simulink model "traiettoria"  (R2022b)
settings: Solver=VariableStepAuto  StartTime=0.0  StopTime=40  RelTol=1e-3
values from neighbouring files (symbols this model uses):
  a1 = W \ [0 0 0.5*pi/2 0]'    [traiettoria_script.m]
  a2 = W \ [0 0 0.25 0]'    [traiettoria_script.m]
  a2_phi = W \ [0 0 pi/2 0]'    [traiettoria_script.m]
  a3 = W \ [0 0 0.25 0]'    [traiettoria_script.m]
  a4 = W \ [0 0 0.5*pi/2 0]'    [traiettoria_script.m]
  a5 = W \ [0 0 0.25 0]'    [traiettoria_script.m]
  a6 = W \ [0 0 0.25 0]'    [traiettoria_script.m]
  a6_phi = W \ [0 0 pi/2 0]'    [traiettoria_script.m]
  a7 = W \ [0 0 0.5*pi/2 0]'    [traiettoria_script.m]
  a8 = W \ [0 0 0.5*pi/2 0]'    [traiettoria_script.m]
  a9 = W \ [0 0 (sqrt(5)/4)*(pi - 2*atan(1/2)) 0]'    [traiettoria_script.m]
  p_d_0 = [0 0.75 -0.25]'    [traiettoria_script.m]
  phi_d_0 = 0    [traiettoria_script.m]
  T = T_A * T_B    [DH_dinamica.m]    (also in traiettoria_script.m = 0.001)
undefined symbols (not defined in the file or in its folder): DiscIntNeverNeededParam
settings Model: Creator=Michele  LastModifiedBy=Michele
settings DataIOCC: ReturnWorkspaceOutputs=off

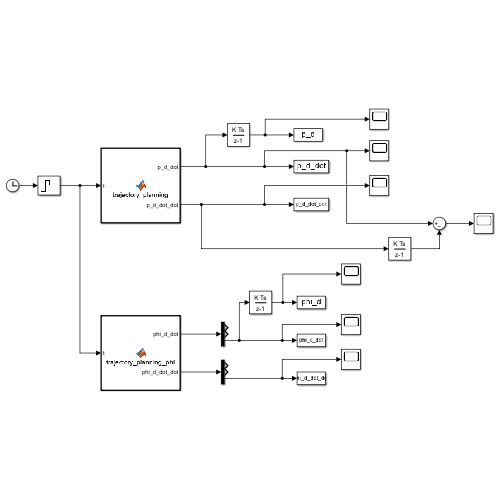
[thumbnail: Simulink's stored preview of the top-level diagram]
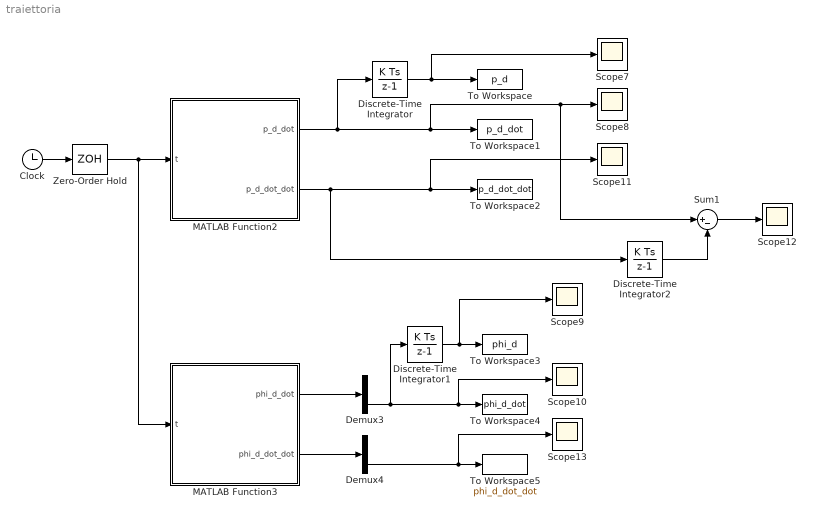
== system traiettoria ==
  Clock : Clock
  Demux3 : Demux  Outputs=3
  Demux4 : Demux  Outputs=3
  Discrete-Time Integrator : DiscreteIntegrator  InitialCondition=p_d_0  SampleTime=-1  ICPrevOutput=DiscIntNeverNeededParam  ICPrevScaledInput=DiscIntNeverNeededParam
  Discrete-Time Integrator1 : DiscreteIntegrator  InitialCondition=phi_d_0  SampleTime=-1  ICPrevOutput=DiscIntNeverNeededParam  ICPrevScaledInput=DiscIntNeverNeededParam
  Discrete-Time Integrator2 : DiscreteIntegrator  InitialCondition=[0 0 0]'  SampleTime=-1  ICPrevOutput=DiscIntNeverNeededParam  ICPrevScaledInput=DiscIntNeverNeededParam
  MATLAB Function2 : MATLAB Function  TreatAsAtomicUnit=on
  MATLAB Function3 : MATLAB Function  TreatAsAtomicUnit=on
  Scope{7..13} (7 alike) : Scope
  Sum1 : Sum  Inputs=|+-
  To Workspace : ToWorkspace  VariableName=p_d  SaveFormat=Structure With Time  SampleTime=-1
      settings: Save2DSignal=2-D array (concatenate along first dimension)
  To Workspace1 : ToWorkspace  VariableName=p_d_dot  SaveFormat=Structure With Time  SampleTime=-1
      settings: Save2DSignal=2-D array (concatenate along first dimension)
  To Workspace2 : ToWorkspace  VariableName=p_d_dot_dot  SaveFormat=Structure With Time  SampleTime=-1
      settings: Save2DSignal=2-D array (concatenate along first dimension)
  To Workspace3 : ToWorkspace  VariableName=phi_d  SaveFormat=Structure With Time  SampleTime=-1
      settings: Save2DSignal=2-D array (concatenate along first dimension)
  To Workspace4 : ToWorkspace  VariableName=phi_d_dot  SaveFormat=Structure With Time  SampleTime=-1
      settings: Save2DSignal=2-D array (concatenate along first dimension)
  To Workspace5 : ToWorkspace  VariableName=phi_d_dot_dot  SaveFormat=Structure With Time  SampleTime=-1
      settings: Save2DSignal=2-D array (concatenate along first dimension)
  Zero-Order Hold : ZeroOrderHold  SampleTime=T
  wires:
  Discrete-Time Integrator/1 -> To Workspace/1, Scope7/1
  Sum1/1 -> Scope12/1
  MATLAB Function2/1(p_d_dot) -> Discrete-Time Integrator/1, Sum1/1, Scope8/1, To Workspace1/1
  MATLAB Function2/2(p_d_dot_dot) -> Discrete-Time Integrator2/1, To Workspace2/1, Scope11/1
  Discrete-Time Integrator2/1 -> Sum1/2
  MATLAB Function3/1(phi_d_dot) -> Demux3/1
  MATLAB Function3/2(phi_d_dot_dot) -> Demux4/1
  Clock/1 -> Zero-Order Hold/1
  Demux3/3 -> Discrete-Time Integrator1/1, Scope10/1, To Workspace4/1
  Discrete-Time Integrator1/1 -> Scope9/1, To Workspace3/1
  Demux4/3 -> Scope13/1, To Workspace5/1
  Zero-Order Hold/1 -> MATLAB Function3/1(t), MATLAB Function2/1(t)

== matlab function traiettoria/MATLAB Function2 ==
  data: t input; a1 parameter; a2 parameter; a3 parameter; p_d_dot output; a4 parameter; a5 parameter; a6 parameter; a7 parameter; a8 parameter; a9 parameter; p_d_dot_dot output
function [p_d_dot,p_d_dot_dot] = trajectory_planning(t, a1, a2, a3, a4, a5, a6, a7, a8, a9)
    if(t<=5)
        s = a1(4)*t^3 + a1(3)*t^2;
        s_dot = 3*a1(4)*t^2 + 2*a1(3)*t;
        s_dot_dot = 6*a1(4)*t + 2*a1(3);
        p_d = [0 0.25 -0.25]' + [0 1 0; 1 0 0; 0 0 -1] * [0.5*cos(s/0.5) 0.5*sin(s/0.5) 0]';
        p_d_dot = [0 1 0; 1 0 0; 0 0 -1] * s_dot * [-sin(s/0.5) cos(s/0.5) 0]';
        p_d_dot_dot = [0 1 0; 1 0 0; 0 0 -1] * (s_dot_dot * [-sin(s/0.5) cos(s/0.5) 0]' + s_dot^2 * [-cos(s/0.5)/0.5 -sin(s/0.5)/0.5 0]');
    elseif(t<=9)
        s = a2(4)*(t-5)^3 + a2(3)*(t-5)^2;
        s_dot = 3*a2(4)*(t-5)^2 + 2*a2(3)*(t-5);
        s_dot_dot = 6*a2(4)*(t-5) + 2*a2(3);
        p_d = [0.5 0.25 -0.25]' + s * [0 0 -1]';
        p_d_dot = s_dot * [0 0 -1]';
        p_d_dot_dot = s_dot_dot * [0 0 -1]';
    elseif(t<=12.5)
        s = a3(4)*(t-9)^3 + a3(3)*(t-9)^2;
        s_dot = 3*a3(4)*(t-9)^2 + 2*a3(3)*(t-9);
        s_dot_dot = 6*a3(4)*(t-9) + 2*a3(3);
        p_d = [0.5 0.25 -0.5]' + s * [0 -1 0]';
        p_d_dot = s_dot * [0 -1 0]';
        p_d_dot_dot = s_dot_dot * [0 -1 0]';
    elseif(t<=13)
        s = a3(4)*(t-9)^3 + a3(3)*(t-9)^2;
        s_dot = 3*a3(4)*(t-9)^2 + 2*a3(3)*(t-9);
        s_dot_dot = 6*a3(4)*(t-9) + 2*a3(3);
        p_d = [0.5 0.25 -0.5]' + s * [0 -1 0]';
        p_d_dot = s_dot * [0 -1 0]';
        p_d_dot_dot = s_dot_dot * [0 -1 0]';

        s = a4(4)*(t-12.5)^3 + a4(3)*(t-12.5)^2;
        s_dot = 3*a4(4)*(t-12.5)^2 + 2*a4(3)*(t-12.5);
        s_dot_dot = 6*a4(4)*(t-12.5) + 2*a4(3);
        p_d = p_d +  [0.5 0.5 -0.5]' + [0 -1 0; -1 0 0; 0 0 -1] * [0.5*cos(s/0.5) 0.5*sin(s/0.5) 0]';
        p_d_dot = p_d_dot + [0 -1 0; -1 0 0; 0 0 -1] * s_dot * [-sin(s/0.5) cos(s/0.5) 0]';
        p_d_dot_dot = p_d_dot_dot + [0 -1 0; -1 0 0; 0 0 -1] * (s_dot_dot * [-sin(s/0.5) cos(s/0.5) 0]' + s_dot^2 * [-cos(s/0.5)/0.5 -sin(s/0.5)/0.5 0]');
    elseif(t<=16.5)
        s = a4(4)*(t-12.5)^3 + a4(3)*(t-12.5)^2;
        s_dot = 3*a4(4)*(t-12.5)^2 + 2*a4(3)*(t-12.5);
        s_dot_dot = 6*a4(4)*(t-12.5) + 2*a4(3);
        p_d = [0.5 0.5 -0.25]' + [0 -1 0; -1 0 0; 0 0 -1] * [0.5*cos(s/0.5) 0.5*sin(s/0.5) 0]';
        p_d_dot = [0 -1 0; -1 0 0; 0 0 -1] * s_dot * [-sin(s/0.5) cos(s/0.5) 0]';
        p_d_dot_dot = [0 -1 0; -1 0 0; 0 0 -1] * (s_dot_dot * [-sin(s/0.5) cos(s/0.5) 0]' + s_dot^2 * [-cos(s/0.5)/0.5 -sin(s/0.5)/0.5 0]');
    elseif(t<=17.5)
        s = a4(4)*(t-12.5)^3 + a4(3)*(t-12.5)^2;
        s_dot = 3*a4(4)*(t-12.5)^2 + 2*a4(3)*(t-12.5);
        s_dot_dot = 6*a4(4)*(t-12.5) + 2*a4(3);
        p_d = [0.5 0.5 -0.5]' + [0 -1 0; -1 0 0; 0 0 -1] * [0.5*cos(s/0.5) 0.5*sin(s/0.5) 0]';
        p_d_dot = [0 -1 0; -1 0 0; 0 0 -1] * s_dot * [-sin(s/0.5) cos(s/0.5) 0]';
        p_d_dot_dot = [0 -1 0; -1 0 0; 0 0 -1] * (s_dot_dot * [-sin(s/0.5) cos(s/0.5) 0]' + s_dot^2 * [-cos(s/0.5)/0.5 -sin(s/0.5)/0.5 0]');

        s = a5(4)*(t-16.5)^3 + a5(3)*(t-16.5)^2;
        s_dot = 3*a5(4)*(t-16.5)^2 + 2*a5(3)*(t-16.5);
        s_dot_dot = 6*a5(4)*(t-16.5) + 2*a5(3);
        p_d = p_d + [0 0.5 -0.5]' + s * [0 1 0]';
        p_d_dot = p_d_dot + s_dot * [0 1 0]';
        p_d_dot_dot = p_d_dot_dot + s_dot_dot * [0 1 0]';
    elseif(t<=20.5)
        s = a5(4)*(t-16.5)^3 + a5(3)*(t-16.5)^2;
        s_dot = 3*a5(4)*(t-16.5)^2 + 2*a5(3)*(t-16.5);
        s_dot_dot = 6*a5(4)*(t-16.5) + 2*a5(3);
        p_d = [0 0.5 -0.5]' + s * [0 1 0]';
        p_d_dot = s_dot * [0 1 0]';
        p_d_dot_dot = s_dot_dot * [0 1 0]';
    elseif(t<=24.5)
        s = a6(4)*(t-20.5)^3 + a6(3)*(t-20.5)^2;
        s_dot = 3*a6(4)*(t-20.5)^2 + 2*a6(3)*(t-20.5);
        s_dot_dot = 6*a6(4)*(t-20.5) + 2*a6(3);
        p_d = [0 0.75 -0.5]' + s * [0 0 1]';
        p_d_dot = s_dot * [0 0 1]';
        p_d_dot_dot = s_dot_dot * [0 0 1]';
    elseif(t<=27)
        s = a7(4)*(t-24.5)^3 + a7(3)*(t-24.5)^2;
        s_dot = 3*a7(4)*(t-24.5)^2 + 2*a7(3)*(t-24.5);
        s_dot_dot = 6*a7(4)*(t-24.5) + 2*a7(3);
        p_d = [0 0.25 0]' + [0 -1 0; 1 0 0; 0 0 1] * [0.5*cos(s/0.5) 0.5*sin(s/0.5) 0]';
        p_d_dot = [0 -1 0; 1 0 0; 0 0 1] * s_dot * [-sin(s/0.5) cos(s/0.5) 0]';
        p_d_dot_dot = [0 -1 0; 1 0 0; 0 0 1] * (s_dot_dot * [-sin(s/0.5) cos(s/0.5) 0]' + s_dot^2 * [-cos(s/0.5)/0.5 -sin(s/0.5)/0.5 0]');
    elseif(t<=28.5)
        s = a7(4)*(t-24.5)^3 + a7(3)*(t-24.5)^2;
        s_dot = 3*a7(4)*(t-24.5)^2 + 2*a7(3)*(t-24.5);
        s_dot_dot = 6*a7(4)*(t-24.5) + 2*a7(3);
        p_d = [0 0.25 -0.25]' + [0 -1 0; 1 0 0; 0 0 1] * [0.5*cos(s/0.5) 0.5*sin(s/0.5) 0]';
        p_d_dot = [0 -1 0; 1 0 0; 0 0 1] * s_dot * [-sin(s/0.5) cos(s/0.5) 0]';
        p_d_dot_dot = [0 -1 0; 1 0 0; 0 0 1] * (s_dot_dot * [-sin(s/0.5) cos(s/0.5) 0]' + s_dot^2 * [-cos(s/0.5)/0.5 -sin(s/0.5)/0.5 0]');

        s = a8(4)*(t-27)^3 + a8(3)*(t-27)^2;
        s_dot = 3*a8(4)*(t-27)^2 + 2*a8(3)*(t-27);
        s_dot_dot = 6*a8(4)*(t-27) + 2*a8(3);
        p_d = p_d + [0 0.25 -0.25]' + [-1 0 0; 0 -1 0; 0 0 1] * [0.5*cos(s/0.5) 0.5*sin(s/0.5) 0]';
        p_d_dot = p_d_dot + [-1 0 0; 0 -1 0; 0 0 1] * s_dot * [-sin(s/0.5) cos(s/0.5) 0]';
        p_d_dot_dot = p_d_dot_dot + [-1 0 0; 0 -1 0; 0 0 1] * (s_dot_dot * [-sin(s/0.5) cos(s/0.5) 0]' + s_dot^2 * [-cos(s/0.5)/0.5 -sin(s/0.5)/0.5 0]');
    elseif(t<=30)
        s = a8(4)*(t-27)^3 + a8(3)*(t-27)^2;
        s_dot = 3*a8(4)*(t-27)^2 + 2*a8(3)*(t-27);
        s_dot_dot = 6*a8(4)*(t-27) + 2*a8(3);
        p_d = [0 0.25 -0.25]' + [-1 0 0; 0 -1 0; 0 0 1] * [0.5*cos(s/0.5) 0.5*sin(s/0.5) 0]';
        p_d_dot = [-1 0 0; 0 -1 0; 0 0 1] * s_dot * [-sin(s/0.5) cos(s/0.5) 0]';
        p_d_dot_dot = [-1 0 0; 0 -1 0; 0 0 1] * (s_dot_dot * [-sin(s/0.5) cos(s/0.5) 0]' + s_dot^2 * [-cos(s/0.5)/0.5 -sin(s/0.5)/0.5 0]');
    elseif(t<=31)
        s = a8(4)*(t-27)^3 + a8(3)*(t-27)^2;
        s_dot = 3*a8(4)*(t-27)^2 + 2*a8(3)*(t-27);
        s_dot_dot = 6*a8(4)*(t-27) + 2*a8(3);
        p_d = [0 0.25 -0.25]' + [-1 0 0; 0 -1 0; 0 0 1] * [0.5*cos(s/0.5) 0.5*sin(s/0.5) 0]';
        p_d_dot = [-1 0 0; 0 -1 0; 0 0 1] * s_dot * [-sin(s/0.5) cos(s/0.5) 0]';
        p_d_dot_dot = [-1 0 0; 0 -1 0; 0 0 1] * (s_dot_dot * [-sin(s/0.5) cos(s/0.5) 0]' + s_dot^2 * [-cos(s/0.5)/0.5 -sin(s/0.5)/0.5 0]');

        s = a9(4)*(t-30)^3 + a9(3)*(t-30)^2;
        s_dot = 3*a9(4)*(t-30)^2 + 2*a9(3)*(t-30);
        s_dot_dot = 6*a9(4)*(t-30) + 2*a9(3);
        p_d = p_d + [-0.25 0.25 -0.25]' + [1 2 0; -2 1 0; 0 0 sqrt(5)]/sqrt(5) * [(sqrt(5)/4)*cos(s/(sqrt(5)/4)) (sqrt(5)/4)*sin(s/(sqrt(5)/4)) 0]';
        p_d_dot = p_d_dot + [1 2 0; -2 1 0; 0 0 sqrt(5)]/sqrt(5) * s_dot * [-sin(s/(sqrt(5)/4)) cos(s/(sqrt(5)/4)) 0]';
        p_d_dot_dot = p_d_dot_dot + [1 2 0; -2 1 0; 0 0 sqrt(5)]/sqrt(5) * (s_dot_dot * [-sin(s/(sqrt(5)/4)) cos(s/(sqrt(5)/4)) 0]' + s_dot^2 * [-cos(s/(sqrt(5)/4))/(sqrt(5)/4) -sin(s/(sqrt(5)/4))/(sqrt(5)/4) 0]');
    elseif(t<=36)
        s = a9(4)*(t-30)^3 + a9(3)*(t-30)^2;
        s_dot = 3*a9(4)*(t-30)^2 + 2*a9(3)*(t-30);
        s_dot_dot = 6*a9(4)*(t-30) + 2*a9(3);
        p_d = [-0.25 0.25 -0.25]' + [1 2 0; -2 1 0; 0 0 sqrt(5)]/sqrt(5) * [(sqrt(5)/4)*cos(s/(sqrt(5)/4)) (sqrt(5)/4)*sin(s/(sqrt(5)/4)) 0]';
        p_d_dot = [1 2 0; -2 1 0; 0 0 sqrt(5)]/sqrt(5) * s_dot * [-sin(s/(sqrt(5)/4)) cos(s/(sqrt(5)/4)) 0]';
        p_d_dot_dot = [1 2 0; -2 1 0; 0 0 sqrt(5)]/sqrt(5) * (s_dot_dot * [-sin(s/(sqrt(5)/4)) cos(s/(sqrt(5)/4)) 0]' + s_dot^2 * [-cos(s/(sqrt(5)/4))/(sqrt(5)/4) -sin(s/(sqrt(5)/4))/(sqrt(5)/4) 0]');
    else
        p_d = [0 0.75 -0.25]';
        p_d_dot = [0 0 0]';
        p_d_dot_dot = [0 0 0]';
    end
end

== matlab function traiettoria/MATLAB Function3 ==
  data: t input; phi_d_dot output; phi_d_dot_dot output; a2_phi parameter; a6_phi parameter
function [phi_d_dot,phi_d_dot_dot] = trajectory_planning_phi(t, a2_phi, a6_phi)
    if(t<=5)
        phi_d = [-pi/2 pi 0];
        phi_d_dot = [0 0 0]';
        phi_d_dot_dot = [0 0 0]';
    elseif(t<=9)
        s = a2_phi(4)*(t-5)^3 + a2_phi(3)*(t-5)^2;
        s_dot = 3*a2_phi(4)*(t-5)^2 + 2*a2_phi(3)*(t-5);
        s_dot_dot = 6*a2_phi(4)*(t-5) + 2*a2_phi(3);
        phi_d = [-pi/2 pi 0]' + s * [0 0 1]';
        phi_d_dot = s_dot * [0 0 1]';
        phi_d_dot_dot = s_dot_dot * [0 0 1]';
    elseif(t<=20.5)
        phi_d = [-pi/2 pi pi/2];
        phi_d_dot = [0 0 0]';
        phi_d_dot_dot = [0 0 0]';
    elseif(t<=24.5)
        s = a6_phi(4)*(t-20.5)^3 + a6_phi(3)*(t-20.5)^2;
        s_dot = 3*a6_phi(4)*(t-20.5)^2 + 2*a6_phi(3)*(t-20.5);
        s_dot_dot = 6*a6_phi(4)*(t-20.5) + 2*a6_phi(3);
        phi_d = [-pi/2 pi pi/2]' + s * [0 0 -1]';
        phi_d_dot = s_dot * [0 0 -1]';
        phi_d_dot_dot = s_dot_dot * [0 0 -1]';
    else
        phi_d = [-pi/2 pi 0];
        phi_d_dot = [0 0 0]';
        phi_d_dot_dot = [0 0 0]';
    end
end
